simulink model "peak_biquad"  (R2018b)
settings: Solver=FixedStepAuto  StartTime=0.0  StopTime=inf  RelTol=1e-3  EnableMultiTasking=on
libraries: stm32f769ilib x2
settings Model: SimulationMode=external  Creator=Pemmavit  LastModifiedBy=hpong
settings OptimizationCC: EnhancedBackFolding=on  PassReuseOutputArgsAs=Individual arguments  MaxStackSize=64  OptimizeBlockOrder=speed  DifferentSizesBufferReuse=on  OptimizationCustomize=off
settings DebuggingCC: ParameterTunabilityLossMsg=error
settings HardwareCC: ProdBitPerPointer=32  ProdBitPerSizeT=32  ProdBitPerPtrDiffT=32  ProdLargestAtomicInteger=Long  ProdLargestAtomicFloat=Double  ProdWordSize=32  ProdHWDeviceType=ARM Compatible->ARM Cortex
settings SFSimCC: MATLABDynamicMemAlloc=off
settings RTWCC: SystemTargetFile=ert.tlc  HardwareBoard=STM32F769I-Discovery  TemplateMakefile=ert_default_tmf  GenerateReport=on  Toolchain=GNU Tools for ARM Embedded Processors  IncludeHyperlinkInReport=on  LaunchReport=on  GenerateTraceInfo=on  GenerateTraceReport=on  GenerateTraceReportSl=on  GenerateTraceReportSf=on  GenerateTraceReportEml=on
settings CodeAppCC: ForceParamTrailComments=on  IgnoreCustomStorageClasses=off  OperatorAnnotations=on  SimulinkDataObjDesc=on  SFDataObjDesc=on  InsertBlockDesc=on
settings ERTTargetCC: CodeReplacementLibrary=ARM Cortex-M (CMSIS)

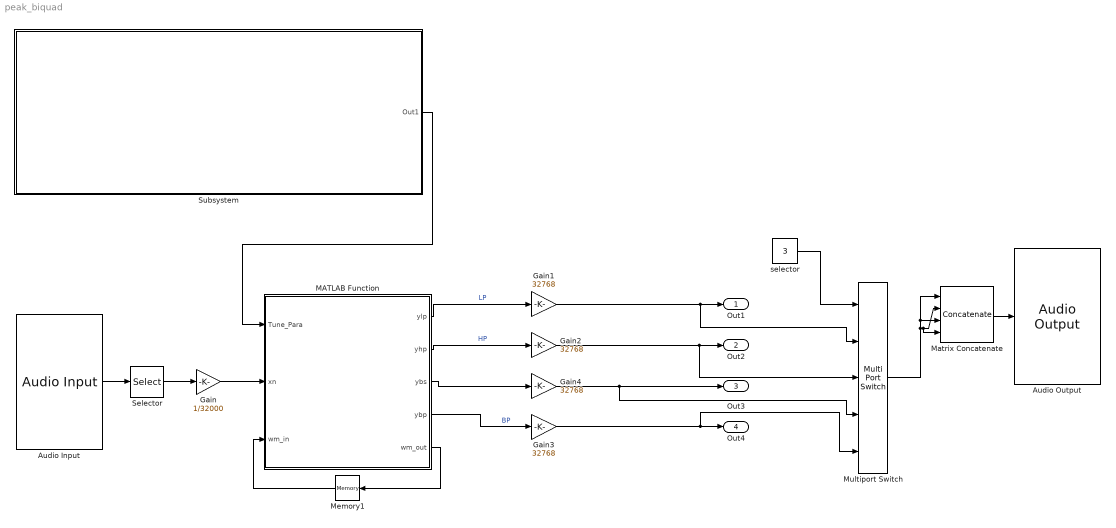
== system peak_biquad ==
  Audio Input : stm32f769ilib/Audio Input  InputDevice=LineIn  SamplingFreq=16000  NumCh=2  FrameSize=4096
      settings: SourceProductName=Embedded Coder Support Package for STMicroelectronics Discovery Boards  SourceProductBaseCode=STMICRODIS
  Audio Output : stm32f769ilib/Audio Output  OutputDevice=Headphone  SamplingFreq=16000  Volume=63
      settings: SourceProductName=Embedded Coder Support Package for STMicroelectronics Discovery Boards  SourceProductBaseCode=STMICRODIS
  Gain : Gain  Gain=1/32000  ParamDataTypeStr=double  OutDataTypeStr=double
  Gain{1..4} (4 alike) : Gain  Gain=32768  ParamDataTypeStr=int16  OutDataTypeStr=int16
  MATLAB Function : MATLAB Function  TreatAsAtomicUnit=on
  Matrix Concatenate : Concatenate  NumInputs=4  Mode=Multidimensional array  ConcatenateDimension=2
  Memory1 : Memory  InitialCondition=[0 0;0 0;0 0;0 0]  InheritSampleTime=on
  Multiport Switch : MultiPortSwitch  Inputs=4
  Selector : Selector  NumberOfDimensions=2  InputPortWidth=3  IndexOptions=Select all,Index vector (dialog)  Indices=[1 3],1  OutputSizes=1,1
  Subsystem : Subsystem
  selector : Constant  Value=3  OutDataTypeStr=int8
  Out1 : Outport  SignalName=LP
  Out2 : Outport  Port=2  SignalName=HP
  Out3 : Outport  Port=3  SignalName=BS
  Out4 : Outport  Port=4  SignalName=BP
  wires:
  Audio Input/1 -> Selector/1
  Selector/1 -> Gain/1
  Matrix Concatenate/1 -> Audio Output/1
  Gain/1 -> MATLAB Function/2(xn)
  MATLAB Function/5(wm_out) -> Memory1/1
  Memory1/1 -> MATLAB Function/3(wm_in)
  MATLAB Function/2(yhp) -> Gain2/1  "HP"
  MATLAB Function/1(ylp) -> Gain1/1  "LP"
  MATLAB Function/4(ybp) -> Gain3/1  "BP"
  Gain1/1 -> Multiport Switch/2, Out1/1
  Gain2/1 -> Multiport Switch/3, Out2/1
  Gain3/1 -> Multiport Switch/5, Out4/1
  Multiport Switch/1 -> Matrix Concatenate/3, Matrix Concatenate/1, Matrix Concatenate/4, Matrix Concatenate/2
  selector/1 -> Multiport Switch/1
  MATLAB Function/3(ybs) -> Gain4/1
  Gain4/1 -> Multiport Switch/4, Out3/1
  Subsystem/1(Out1) -> MATLAB Function/1(Tune_Para)

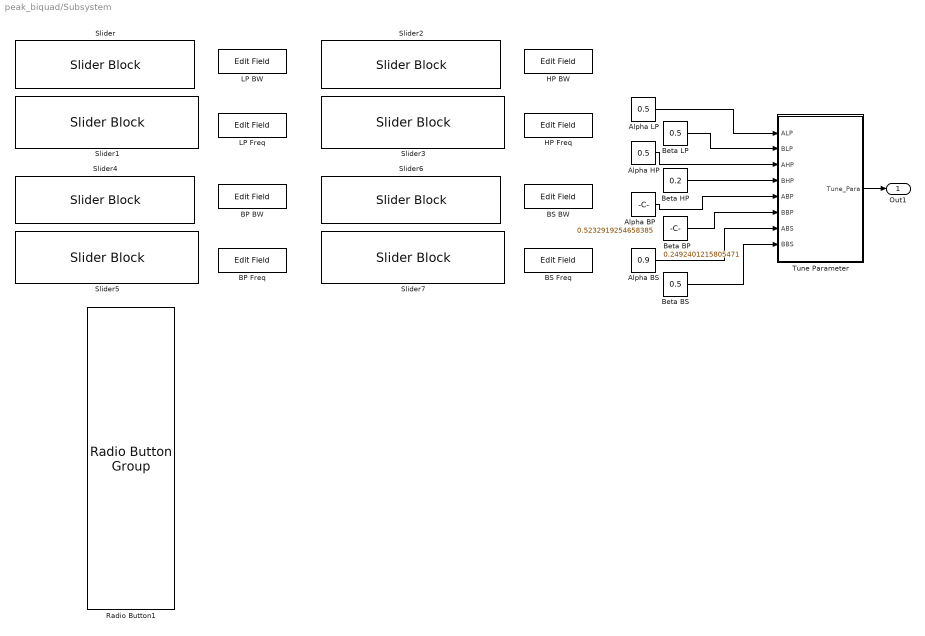
== system peak_biquad/Subsystem ==
  Alpha BP : Constant  Value=0.5232919254658385
  Alpha BS : Constant  Value=0.9
  Alpha HP : Constant  Value=0.5
  Alpha LP : Constant  Value=0.5
  BP BW : EditField  WebBlockId=46  LabelPosition=Hide  ShowInitialText=on  Alignment=Center
  BP Freq : EditField  WebBlockId=47  LabelPosition=Hide  ShowInitialText=on  Alignment=Center
  BS BW : EditField  WebBlockId=48  LabelPosition=Hide  ShowInitialText=on  Alignment=Center
  BS Freq : EditField  WebBlockId=49  LabelPosition=Hide  ShowInitialText=on  Alignment=Center
  Beta BP : Constant  Value=0.2492401215805471
  Beta BS : Constant  Value=0.5
  Beta HP : Constant  Value=0.2
  Beta LP : Constant  Value=0.5
  HP BW : EditField  WebBlockId=39  LabelPosition=Hide  ShowInitialText=on  Alignment=Center
  HP Freq : EditField  WebBlockId=40  LabelPosition=Hide  ShowInitialText=on  Alignment=Center
  LP BW : EditField  WebBlockId=14  LabelPosition=Hide  ShowInitialText=on  Alignment=Center
  LP Freq : EditField  WebBlockId=15  LabelPosition=Hide  ShowInitialText=on  Alignment=Center
  Radio Button1 : RadioButtonGroup  WebBlockId=38  SelectedLabel=BS  ButtonGroupName=Group
      settings: Values={{'LP', 'HP', 'BS', 'BP'}, [1 2 3 4]}
  Slider : SliderBlock  WebBlockId=35  ScaleMax=1
  Slider1 : SliderBlock  WebBlockId=36  ScaleMax=1
  Slider2 : SliderBlock  WebBlockId=41  ScaleMax=1
  Slider3 : SliderBlock  WebBlockId=42  ScaleMax=1
  Slider4 : SliderBlock  WebBlockId=50  ScaleMax=1
  Slider5 : SliderBlock  WebBlockId=51  ScaleMax=1
  Slider6 : SliderBlock  WebBlockId=52  ScaleMax=1
  Slider7 : SliderBlock  WebBlockId=53  ScaleMax=1
  Tune Parameter : MATLAB Function  TreatAsAtomicUnit=on
  Out1 : Outport
  wires:
  Alpha LP/1 -> Tune Parameter/1(ALP)
  Beta LP/1 -> Tune Parameter/2(BLP)
  Alpha HP/1 -> Tune Parameter/3(AHP)
  Beta HP/1 -> Tune Parameter/4(BHP)
  Alpha BP/1 -> Tune Parameter/5(ABP)
  Beta BP/1 -> Tune Parameter/6(BBP)
  Alpha BS/1 -> Tune Parameter/7(ABS)
  Beta BS/1 -> Tune Parameter/8(BBS)
  Tune Parameter/1(Tune_Para) -> Out1/1

== matlab function peak_biquad/Subsystem/Tune Parameter ==
  data: ALP input; Tune_Para output; BLP input; AHP input; BHP input; ABP input; BBP input; ABS input; BBS input
function Tune_Para = fcn(ALP,BLP,AHP,BHP,ABP,BBP,ABS,BBS)

Tune_Para = [ALP cos(BLP*pi);AHP cos(BHP*pi);ABS cos(BBS*pi);ABP cos(BBP*pi)];

== matlab function peak_biquad/MATLAB Function ==
  data: Tune_Para input; ylp output; yhp output; ybs output; xn input; ybp output; wm_in input; wm_out output
function [ylp, yhp,  ybs,ybp, wm_out] = iir_test(Tune_Para, xn,wm_in)
sample_per_frame = 4096;

wn = ones(4,3); d1 = ones(4,1); d2  = ones(4,1); Glp = ones(4,1); Ghp = ones(4,1); Gbp = ones(4,1);
ylp = ones(sample_per_frame,1,'double');
yhp = ylp;
ybp = ylp;
ybs = ylp;
wn(:,2:3) = wm_in;

for i=1:4   % 1 = alpha     2 = Beta
    d1(i) = -(1+Tune_Para(i,1))*Tune_Para(i,2);
    d2(i) = Tune_Para(i,1);
    Glp(i) = 0.25*(1-Tune_Para(i,2))*(1+Tune_Para(i,1));
    Ghp(i) = 0.25*(1+Tune_Para(i,2))*(1+Tune_Para(i,1));
    Gbp(i) = 0.5*(1-Tune_Para(i,1));
end

for i=1:4 %1=LP     2=HP      3=BS     4=BP
    for n = 1:sample_per_frame
        wn(i,1) = xn(n) - wn(i,2)*d1(i) - wn(i,3)*d2(i);
        switch i
            case 1
                ylp(n) = (wn(i,1) + wn(i,3) + 2*wn(i,2))*Glp(i);
            case 2
                yhp(n) = (wn(i,1) + wn(i,3) - 2*wn(i,2))*Ghp(i);
            case 4
                ybp(n) = (wn(i,1) - wn(i,3))*Gbp(i);
            case 3
                ybs(n) = (wn(i,1) + wn(i,3) + 2*wn(i,2))*Glp(i) + (wn(i,1) + wn(i,3) - 2*wn(i,2))*Ghp(i)+(wn(i,1) - wn(i,3))*Gbp(i)*3;
        end
        wn(i,3) = wn(i,2);
        wn(i,2) = wn(i,1);
    end
end
wm_out = wn(:,1:2);
%-------------------------------------------
